simulink model "LQR"  (R2022b)
settings: Solver=VariableStepAuto  StartTime=0.0  StopTime=10.0  RelTol=1e-3
settings Model: Creator=zhouwenjie  LastModifiedBy=zhouwenjie

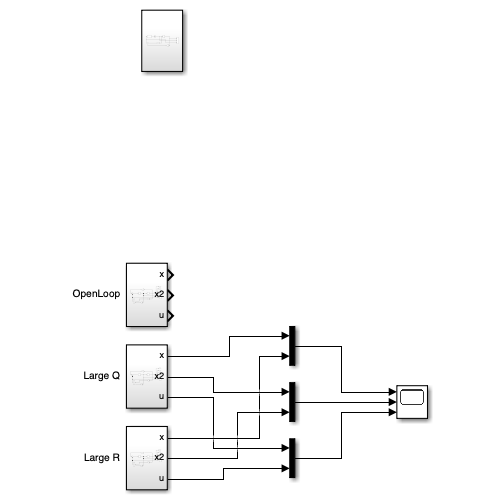
[thumbnail: Simulink's stored preview of the top-level diagram]
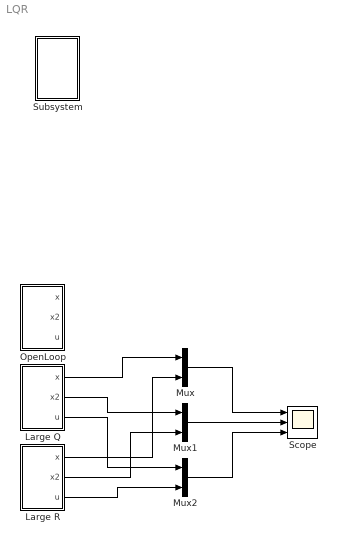
== system LQR ==
  Large Q : Subsystem
  Large R : Subsystem
  Mux : Mux  Inputs=2
  Mux1 : Mux  Inputs=2
  Mux2 : Mux  Inputs=2
  OpenLoop : Subsystem
  Scope : Scope  NumInputPorts=3
  Subsystem : Subsystem
  wires:
  Large Q/1(x) -> Mux/1
  Large R/1(x) -> Mux/2
  Large Q/2(x2) -> Mux1/1
  Large Q/3(u) -> Mux2/1
  Large R/2(x2) -> Mux1/2
  Large R/3(u) -> Mux2/2
  Mux/1 -> Scope/1
  Mux1/1 -> Scope/2
  Mux2/1 -> Scope/3

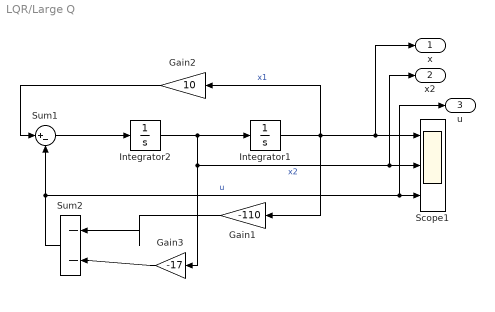
== system LQR/Large Q ==
  Gain1 : Gain  Gain=-110
  Gain2 : Gain  Gain=10
  Gain3 : Gain  Gain=-17
  Integrator1 : Integrator  InitialCondition=5
  Integrator2 : Integrator
  Scope1 : Scope  NumInputPorts=3
  Sum1 : Sum  Inputs=|+-
  Sum2 : Sum  Inputs=|--
  x : Outport
  x2 : Outport  Port=2
  u : Outport  Port=3
  wires:
  Integrator2/1 -> Integrator1/1, Scope1/2, x2/1, Gain3/1  "x2"
  Gain1/1 -> Sum2/1
  Sum2/1 -> Scope1/3, u/1, Sum1/2  "u"
  Integrator1/1 -> Scope1/1, x/1, Gain2/1, Gain1/1  "x1"
  Gain3/1 -> Sum2/2
  Sum1/1 -> Integrator2/1
  Gain2/1 -> Sum1/1

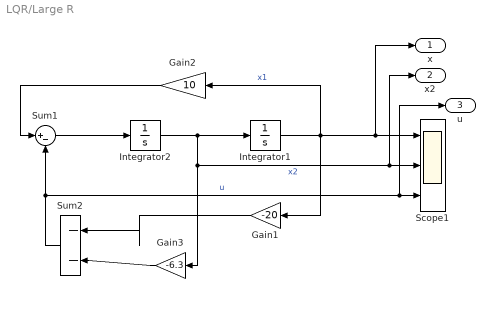
== system LQR/Large R ==
  Gain1 : Gain  Gain=-20
  Gain2 : Gain  Gain=10
  Gain3 : Gain  Gain=-6.3
  Integrator1 : Integrator  InitialCondition=5
  Integrator2 : Integrator
  Scope1 : Scope  NumInputPorts=3
  Sum1 : Sum  Inputs=|+-
  Sum2 : Sum  Inputs=|--
  x : Outport
  x2 : Outport  Port=2
  u : Outport  Port=3
  wires:
  Gain2/1 -> Sum1/1
  Sum1/1 -> Integrator2/1
  Gain3/1 -> Sum2/2
  Integrator1/1 -> Gain1/1, Gain2/1, x/1, Scope1/1  "x1"
  Sum2/1 -> Sum1/2, u/1, Scope1/3  "u"
  Gain1/1 -> Sum2/1
  Integrator2/1 -> Gain3/1, x2/1, Scope1/2, Integrator1/1  "x2"

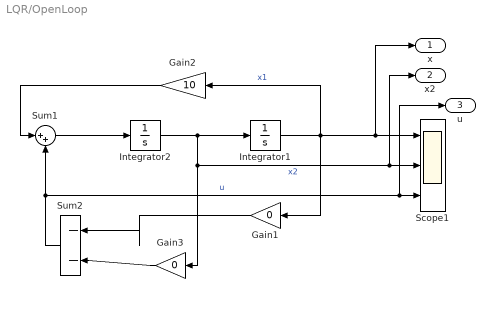
== system LQR/OpenLoop ==
  Gain1 : Gain  Gain=0
  Gain2 : Gain  Gain=10
  Gain3 : Gain  Gain=0
  Integrator1 : Integrator  InitialCondition=1
  Integrator2 : Integrator
  Scope1 : Scope  NumInputPorts=3
  Sum1 : Sum  Inputs=|++
  Sum2 : Sum  Inputs=|--
  x : Outport
  x2 : Outport  Port=2
  u : Outport  Port=3
  wires:
  Gain2/1 -> Sum1/1
  Sum1/1 -> Integrator2/1
  Gain3/1 -> Sum2/2
  Integrator1/1 -> Gain1/1, Gain2/1, x/1, Scope1/1  "x1"
  Sum2/1 -> Sum1/2, u/1, Scope1/3  "u"
  Gain1/1 -> Sum2/1
  Integrator2/1 -> Gain3/1, x2/1, Scope1/2, Integrator1/1  "x2"

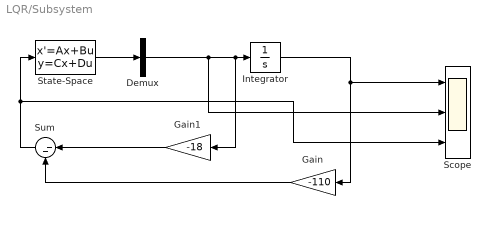
== system LQR/Subsystem ==
  Demux : Demux  Outputs=1
  Gain : Gain  Gain=-110
  Gain1 : Gain  Gain=-18
  Integrator : Integrator
  Scope : Scope  NumInputPorts=3
  State-Space : StateSpace  A=[0 1;10 0]  B=[0;-1]  C=[0 1]  D=[0]  InitialCondition=5
  Sum : Sum  Inputs=|--
  wires:
  Sum/1 -> Scope/3, State-Space/1
  Demux/1 -> Scope/2, Gain1/1, Integrator/1
  Gain/1 -> Sum/2
  State-Space/1 -> Demux/1
  Integrator/1 -> Scope/1, Gain/1
  Gain1/1 -> Sum/1
